simulink model "LTI_Lon_and_Lat_missile"  (R2022b)
settings: Solver=VariableStepAuto  StartTime=0.0  StopTime=10  RelTol=1e-3
InitFcn:
  | clear, close all
  | load Llinear_Model.mat
values from neighbouring files (symbols this model uses):
  A_lat = zeros( 4, 4 )    [Lin_Main_missile.m]    (also in Llinear_Model.mat = [-3.4885247997 -0.0131551980639 0.0687754319225 0 8.04005968)
  A_long = zeros( 4, 4 )    [Lin_Main_missile.m]    (also in Llinear_Model.mat = [-0.0691611627081 -0.146012983237 0.0911103138725 0 0.002592)
  B_lat = zeros( 4, 2 )    [Lin_Main_missile.m]    (also in Llinear_Model.mat = [-5.7101610929e-33  155.027070182; 0  0; 1.81304404257e-20  )
  B_long = [ B(Idx_U,2), B(Idx_W,2), B(Idx_Q,2), B(Idx_THETA,2) ]'    [Lin_Main_missile.m]    (also in Llinear_Model.mat = [0 0 0 0])
  C_lat = zeros( 4, 4 )    [Lin_Main_missile.m]    (also in Llinear_Model.mat = [1 0 0 0 0 1 0 0 0 0 1 0 ... (16 elements, 4x4)])
  C_long = zeros( 4, 4 )    [Lin_Main_missile.m]    (also in Llinear_Model.mat = [1 0 0 0 0 1 0 0 0 0 1 0 ... (16 elements, 4x4)])
  D_lat = zeros( 4, 2 )    [Lin_Main_missile.m]    (also in Llinear_Model.mat = [0  0; 0  0; 0  0; 0  0])
  D_long = [ D(Idx_U,2), D(Idx_W,2), D(Idx_Q,2), D(Idx_THETA,2) ]'    [Lin_Main_missile.m]    (also in Llinear_Model.mat = [0 0 0 0])
libraries: simulink_extras x8
settings Model: Creator=Komsun  LastModifiedBy=Komsun

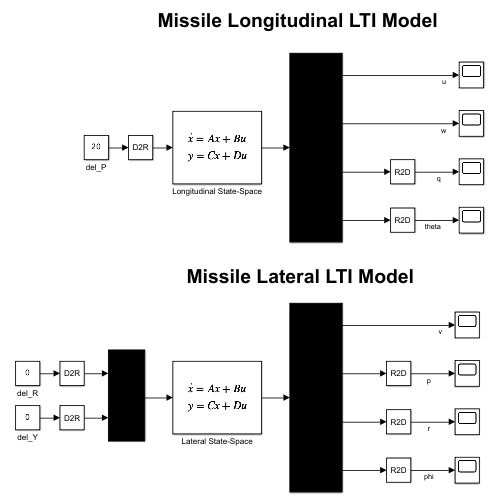
[thumbnail: Simulink's stored preview of the top-level diagram]
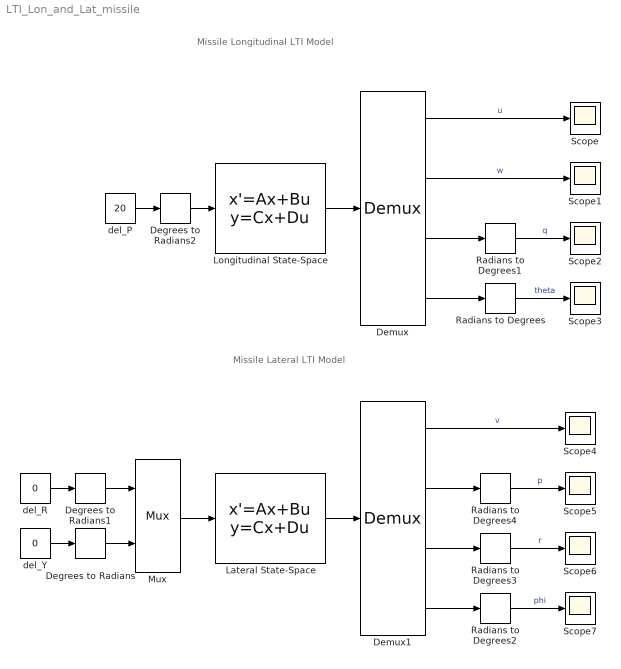
== system LTI_Lon_and_Lat_missile ==
  note: Missile Longitudinal LTI Model
  note: Missile Lateral LTI Model
  Degrees to Radians : simulink_extras/Transformations/Degrees to Radians
  Degrees to Radians1 : simulink_extras/Transformations/Degrees to Radians
  Degrees to Radians2 : simulink_extras/Transformations/Degrees to Radians
  Demux : Demux
  Demux1 : Demux
  Lateral State-Space : StateSpace  A=A_lat  B=B_lat  C=C_lat  D=D_lat  InitialCondition=[0 200*pi/180 0 0]
  Longitudinal State-Space : StateSpace  A=A_long  B=B_long  C=C_long  D=D_long  InitialCondition=[20 0 0 0]
  Mux : Mux  Inputs=2
  Radians to Degrees{,1..4} (5 alike) : simulink_extras/Transformations/Radians to Degrees
  Scope{,1..7} (8 alike) : Scope
  del_P : Constant  Value=20
  del_R : Constant  Value=0
  del_Y : Constant  Value=0
  wires:
  del_P/1 -> Degrees to Radians2/1
  Longitudinal State-Space/1 -> Demux/1
  Demux/1 -> Scope/1  "u"
  Demux/2 -> Scope1/1  "w"
  Demux/3 -> Radians to Degrees1/1
  Demux/4 -> Radians to Degrees/1
  Radians to Degrees/1 -> Scope3/1  "theta"
  Radians to Degrees1/1 -> Scope2/1  "q"
  Radians to Degrees3/1 -> Scope6/1  "r"
  Lateral State-Space/1 -> Demux1/1
  Demux1/1 -> Scope4/1  "v"
  Demux1/2 -> Radians to Degrees4/1
  Demux1/4 -> Radians to Degrees2/1
  Radians to Degrees2/1 -> Scope7/1  "phi"
  Demux1/3 -> Radians to Degrees3/1
  Radians to Degrees4/1 -> Scope5/1  "p"
  Mux/1 -> Lateral State-Space/1
  del_R/1 -> Degrees to Radians1/1
  del_Y/1 -> Degrees to Radians/1
  Degrees to Radians/1 -> Mux/2
  Degrees to Radians1/1 -> Mux/1
  Degrees to Radians2/1 -> Longitudinal State-Space/1
